simulink model "Sistema"  (R2023a)
settings: Solver=ode23  StartTime=0.0  StopTime=10.0  MaxStep=1E-3  RelTol=1e-3
libraries: slpidlib x1
settings Model: Creator=HP  LastModifiedBy=Miria
settings OptimizationCC: ReuseModelBlockBuffer=off
settings DebuggingCC: UnconnectedInputMsg=warning  UnconnectedOutputMsg=warning  UnconnectedLineMsg=warning
settings ModelReferenceCC: EnableRefExpFcnMdlSchedulingChecks=on
settings RTWCC: DLArmComputeVersion=19.05

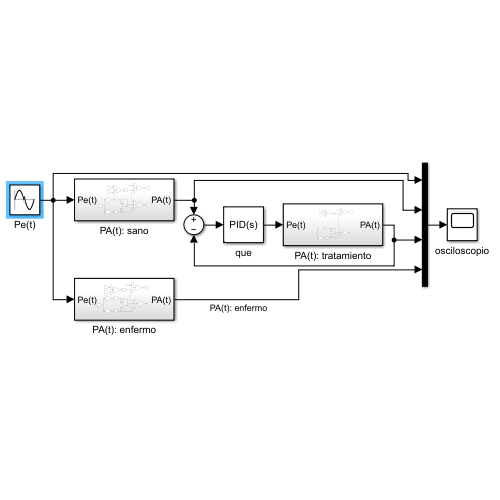
[thumbnail: Simulink's stored preview of the top-level diagram]
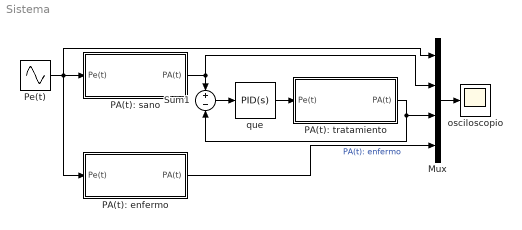
== system Sistema ==
  Mux : Mux
  PA(t): enfermo : Subsystem
  PA(t): sano : Subsystem
  PA(t): tratamiento : Subsystem
  Pe(t) : Sin  Frequency=1.5  SampleTime=0
  Sum1 : Sum  Inputs=+-
  osciloscopio : Scope
  que : slpidlib/PID Controller  Controller=PID  Form=Parallel  TimeDomain=Continuous-time  UseExternalTs=off  SampleTime=-1  IntegratorMethod=Forward Euler  FilterMethod=Forward Euler  ControllerParametersSource=internal  P=195138.40969661  I=16820975.3611442  UseKiTs=off  D=555.656676602032  N=1  UseFilter=on  TunerSelectOption=Transfer Function Based (PID Tuner App)  InitialConditionSource=internal  InitialConditionForIntegrator=0  InitialConditionForFilter=0  DifferentiatorICPrevScaledInput=0  ExternalReset=none  TrackingMode=off  Kt=1  LimitOutput=off  SatLimitsSource=internal  UpperSaturationLimit=inf  LowerSaturationLimit=-inf  LinearizeAsGain=on  AntiWindupMode=none  Kb=1  LimitIntegrator=off  UpperIntegratorSaturationLimit=inf  LowerIntegratorSaturationLimit=-inf  POutMin=[]  POutMax=[]  IOutMin=[]  IOutMax=[]  DOutMin=[]  DOutMax=[]  NOutMin=[]  NOutMax=[]  SumOutMin=[]  SumOutMax=[]  SaturationOutMin=[]  SaturationOutMax=[]  PParamMin=[]  PParamMax=[]  IParamMin=[]  IParamMax=[]  DParamMin=[]  DParamMax=[]  NParamMin=[]  NParamMax=[]  KbParamMin=[]  KbParamMax=[]  KtParamMin=[]  KtParamMax=[]  KbOutMin=[]  KbOutMax=[]  KtOutMin=[]  KtOutMax=[]  IntegratorOutMin=[]  IntegratorOutMax=[]  FilterOutMin=[]  FilterOutMax=[]  SumI1OutMin=[]  SumI1OutMax=[]  SumI2OutMin=[]  SumI2OutMax=[]  SumI3OutMin=[]  SumI3OutMax=[]  SumI4OutMin=[]  SumI4OutMax=[]  SumDOutMin=[]  SumDOutMax=[]  DifferentiatorOutMin=[]  DifferentiatorOutMax=[]  FilterDiffOutCoefMin=[]  FilterDiffOutCoefMax=[]  ReciprocalOutMin=[]  ReciprocalOutMax=[]  SumDenOutMin=[]  SumDenOutMax=[]  SumNumOutMin=[]  SumNumOutMax=[]  DivideOutMin=[]  DivideOutMax=[]  UdiffTsProdOutMin=[]  UdiffTsProdOutMax=[]  NTsProdOutMin=[]  NTsProdOutMax=[]  UintegralTsProdOutMin=[]  UintegralTsProdOutMax=[]  UngainTsProdOutMin=[]  UngainTsProdOutMax=[]  ClampingZeroOutDataTypeStr=Inherit: Inherit via back propagation  ClampingZeroOutMin=[]  ClampingZeroOutMax=[]  FilterDenConstantOutDataTypeStr=Inherit: Inherit via back propagation  FilterDenConstantOutMin=[]  FilterDenConstantOutMax=[]  PCopyOutDataTypeStr=Inherit: Inherit via back propagation  PCopyOutMin=[]  PCopyOutMax=[]  NCopyOutDataTypeStr=Inherit: Inherit via back propagation  NCopyOutMin=[]  NCopyOutMax=[]  IntegratorContinuousStateAttributes=''  IntegratorStateMustResolveToSignalObject=off  IntegratorRTWStateStorageClass=Auto  FilterContinuousStateAttributes=''  FilterStateMustResolveToSignalObject=off  FilterRTWStateStorageClass=Auto  ParallelPVariant=InternalParameters  IdealPVariant=Disabled  IVariant=InternalParameters  DVariant=InternalParameters  IntegratorVariant=Continuous  SatVariant=Disabled  AWVariant=Passthrough  PCopyVariant=Disabled  TRVariant=Disabled  FdbkBlocksVariant=Forward  IdealPFdbkVariant=Disabled  SatFdbkVariant=Disabled  DerivativeFilterVariant=ContFilter  NVariant=InternalParameters  NCopyVariant=Disabled  FilterICVariant=InternalICsFilter  IntegratorICVariant=InternalICs  ExternalResetVariant=Disabled  TRSumVariant=Passthrough  SumFdbkVariant=Disabled  SumVariant=Sum_PID  TsampFilterVariant=InternalTs  TsampNgainVariant=Passthrough  TsampIntegralVariant=Disabled_SignalSpec  ExternalSaturationOutDataTypeStr=Inherit: Same as second input
  wires:
  Mux/1 -> osciloscopio/1
  Sum1/1 -> que/1
  Pe(t)/1 -> PA(t): enfermo/1(Pe(t)), PA(t): sano/1(Pe(t)), Mux/1
  PA(t): enfermo/1(PA(t)) -> Mux/4  "PA(t): enfermo"
  PA(t): sano/1(PA(t)) -> Mux/2, Sum1/1
  que/1 -> PA(t): tratamiento/1(Pe(t))
  PA(t): tratamiento/1(PA(t)) -> Mux/3, Sum1/2

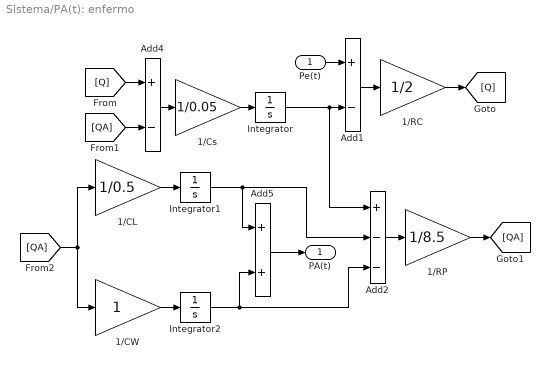
== system Sistema/PA(t): enfermo ==
  Pe(t) : Inport
  1/CL : Gain  Gain=1/0.5
  1/CW : Gain
  1/Cs : Gain  Gain=1/0.05
  1/RC : Gain  Gain=1/2
  1/RP : Gain  Gain=1/8.5
  Add1 : Sum  Inputs=+-
  Add2 : Sum  Inputs=+--
  Add4 : Sum  Inputs=+-
  Add5 : Sum
  Integrator : Integrator
  Integrator1 : Integrator
  Integrator2 : Integrator
  PA(t) : Outport
  wires:
  1/RC/1 -> [Q]
  Add1/1 -> 1/RC/1
  1/RP/1 -> [QA]
  Add2/1 -> 1/RP/1
  [Q] -> Add4/1
  [QA] -> Add4/2
  Add4/1 -> 1/Cs/1
  1/Cs/1 -> Integrator/1
  Pe(t)/1 -> Add1/1
  [QA] -> 1/CL/1, 1/CW/1
  1/CL/1 -> Integrator1/1
  1/CW/1 -> Integrator2/1
  Add5/1 -> PA(t)/1
  Integrator2/1 -> Add5/2, Add2/3
  Integrator/1 -> Add2/1, Add1/2
  Integrator1/1 -> Add5/1, Add2/2

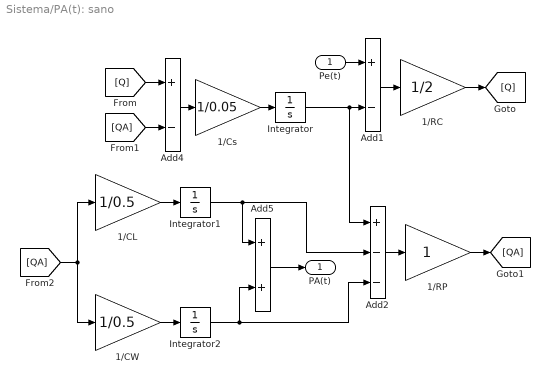
== system Sistema/PA(t): sano ==
  Pe(t) : Inport
  1/CL : Gain  Gain=1/0.5
  1/CW : Gain  Gain=1/0.5
  1/Cs : Gain  Gain=1/0.05
  1/RC : Gain  Gain=1/2
  1/RP : Gain
  Add1 : Sum  Inputs=+-
  Add2 : Sum  Inputs=+--
  Add4 : Sum  Inputs=+-
  Add5 : Sum
  Integrator : Integrator
  Integrator1 : Integrator
  Integrator2 : Integrator
  PA(t) : Outport
  wires:
  1/RC/1 -> [Q]
  Add1/1 -> 1/RC/1
  1/RP/1 -> [QA]
  Add2/1 -> 1/RP/1
  [Q] -> Add4/1
  [QA] -> Add4/2
  Add4/1 -> 1/Cs/1
  1/Cs/1 -> Integrator/1
  Pe(t)/1 -> Add1/1
  [QA] -> 1/CL/1, 1/CW/1
  1/CL/1 -> Integrator1/1
  1/CW/1 -> Integrator2/1
  Add5/1 -> PA(t)/1
  Integrator2/1 -> Add5/2, Add2/3
  Integrator/1 -> Add2/1, Add1/2
  Integrator1/1 -> Add5/1, Add2/2

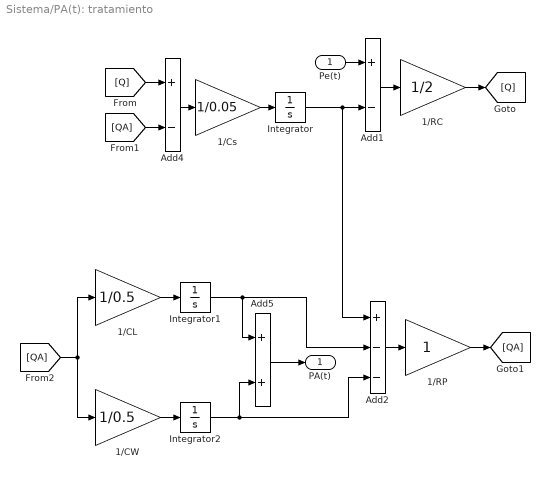
== system Sistema/PA(t): tratamiento ==
  Pe(t) : Inport
  1/CL : Gain  Gain=1/0.5
  1/CW : Gain  Gain=1/0.5
  1/Cs : Gain  Gain=1/0.05
  1/RC : Gain  Gain=1/2
  1/RP : Gain
  Add1 : Sum  Inputs=+-
  Add2 : Sum  Inputs=+--
  Add4 : Sum  Inputs=+-
  Add5 : Sum
  Integrator : Integrator
  Integrator1 : Integrator
  Integrator2 : Integrator
  PA(t) : Outport
  wires:
  1/RC/1 -> [Q]
  Add1/1 -> 1/RC/1
  1/RP/1 -> [QA]
  Add2/1 -> 1/RP/1
  [Q] -> Add4/1
  [QA] -> Add4/2
  Add4/1 -> 1/Cs/1
  1/Cs/1 -> Integrator/1
  Pe(t)/1 -> Add1/1
  [QA] -> 1/CL/1, 1/CW/1
  1/CL/1 -> Integrator1/1
  1/CW/1 -> Integrator2/1
  Add5/1 -> PA(t)/1
  Integrator2/1 -> Add5/2, Add2/3
  Integrator/1 -> Add2/1, Add1/2
  Integrator1/1 -> Add5/1, Add2/2
